simulink library "ctl_controller"  (R2016b)
settings: Solver=ode45  StartTime=0.0  StopTime=10.0  RelTol=1e-3  EnableMultiTasking=on
values from neighbouring files (symbols this model uses):
  ctl_ts = astrobee_fsw_step_size    [ctl_controller_init.m]
undefined symbols (not defined in the file or in its folder): astrobee_fsw_step_size, est_omega_B_ISS_B, est_V_B_ISS_ISS, tun_debug_ctl_use_truth
undefined symbols (not defined in the file): tun_truth_velocity_filt_cutoff_freq, tun_truth_velocity_filt_enable
libraries: math_utils x2, cex_control_executive_lib x1, clc_closed_loop_controller_lib x1, cmd_command_shaper_lib x1, simulink x1
settings Model: Creator=mjmcinty  LastModifiedBy=jfusco1
settings DataIOCC: LimitDataPoints=on  SaveFormat=Array
settings OptimizationCC: LifeSpan=inf
settings DebuggingCC: SolverPrmCheckMsg=warning  AllowSymbolicDim=off  SFUnexpectedBacktrackingDiag=warning  SFNoUnconditionalDefaultTransitionDiag=warning  SFExecutionAtInitializationDiag=none
settings HardwareCC: ProdBitPerPointer=32  ProdBitPerSizeT=32  ProdBitPerPtrDiffT=32  ProdLargestAtomicFloat=None  ProdIntDivRoundTo=Undefined  ProdEndianess=Unspecified  ProdWordSize=32  ProdHWDeviceType=32-bit Generic
settings ModelReferenceCC: PropagateSignalLabelsOutOfModel=off
settings GRTTargetCC: TargetLangStandard=C89/C90 (ANSI)  GeneratePreprocessorConditionals=Disable all
settings ConfigComp: CovMetricSettings=dw  CovHtmlReporting=on  CovSaveCumulativeToWorkspaceVar=on  CovSaveSingleToWorkspaceVar=on  CovExternalEMLEnable=off  CovSFcnEnable=off

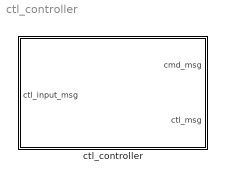
== system ctl_controller ==
  ctl_controller : Subsystem  TreatAsAtomicUnit=on  SystemSampleTime=ctl_ts

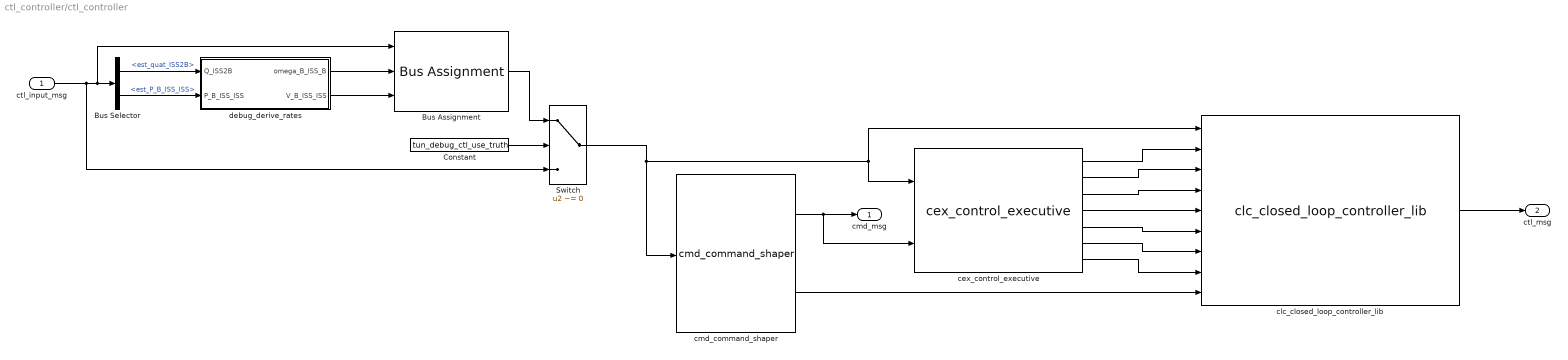
== system ctl_controller/ctl_controller ==
  ctl_input_msg : Inport  OutDataTypeStr=Bus: ctl_input_msg
  Bus Assignment : BusAssignment  AssignedSignals=est_omega_B_ISS_B,est_V_B_ISS_ISS
  Bus Selector : BusSelector  OutputSignals=est_quat_ISS2B,est_P_B_ISS_ISS
  Constant : Constant  Value=tun_debug_ctl_use_truth
  Switch : Switch  Criteria=u2 ~= 0
  cex_control_executive : cex_control_executive_lib/cex_control_executive
  clc_closed_loop_controller_lib : clc_closed_loop_controller_lib/clc_closed_loop_controller_lib
  cmd_command_shaper : cmd_command_shaper_lib/cmd_command_shaper
  debug_derive_rates : Subsystem
  cmd_msg : Outport
  ctl_msg : Outport  Port=2
  wires:
  ctl_input_msg/1 -> Switch/3, Bus Assignment/1, Bus Selector/1
  Bus Assignment/1 -> Switch/1
  Constant/1 -> Switch/2
  clc_closed_loop_controller_lib/1 -> ctl_msg/1
  cex_control_executive/5 -> clc_closed_loop_controller_lib/6
  cex_control_executive/4 -> clc_closed_loop_controller_lib/5
  cex_control_executive/3 -> clc_closed_loop_controller_lib/4
  cex_control_executive/2 -> clc_closed_loop_controller_lib/3
  cex_control_executive/1 -> clc_closed_loop_controller_lib/2
  cmd_command_shaper/1 -> cmd_msg/1, cex_control_executive/2
  Switch/1 -> cmd_command_shaper/1, cex_control_executive/1, clc_closed_loop_controller_lib/1
  cex_control_executive/6 -> clc_closed_loop_controller_lib/7
  cmd_command_shaper/2 -> clc_closed_loop_controller_lib/9
  cex_control_executive/7 -> clc_closed_loop_controller_lib/8
  Bus Selector/1 -> debug_derive_rates/1(Q_ISS2B)  "<est_quat_ISS2B>"
  Bus Selector/2 -> debug_derive_rates/2(P_B_ISS_ISS)  "<est_P_B_ISS_ISS>"
  debug_derive_rates/1(omega_B_ISS_B) -> Bus Assignment/2
  debug_derive_rates/2(V_B_ISS_ISS) -> Bus Assignment/3

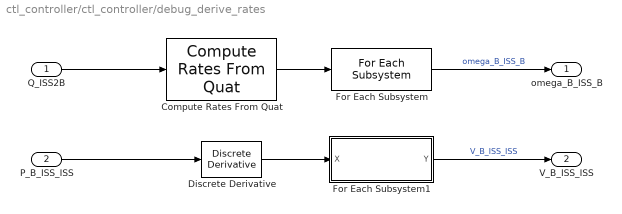
== system ctl_controller/ctl_controller/debug_derive_rates ==
  Q_ISS2B : Inport
  P_B_ISS_ISS : Inport  Port=2
  Compute Rates From Quat : math_utils/Compute Rates From Quat  SystemSampleTime=-1
  Discrete Derivative : simulink/Discrete/Discrete Derivative  gainval=1.0  ICPrevScaledInput=0.0  OutMin=[]  OutMax=[]  OutDataType=fixdt(1, 16)  OutScaling=2^-10  DoSatur=off
  For Each Subsystem : math_utils/For Each Subsystem  T=astrobee_fsw_step_size  omega=tun_truth_q_omega_filt_cutoff_freq  filt_enable=tun_truth_q_omega_filt_enable
  For Each Subsystem1 : Subsystem  TreatAsAtomicUnit=on  mask{T=astrobee_fsw_step_size, omega=tun_truth_velocity_filt_cutoff_freq, filt_enable=tun_truth_velocity_filt_enable}
      mask prompts: T "Sample Time:"; omega "Cutoff Freq (rad/sec):"; filt_enable "Enable Filter:"
      mask DialogControl DescTextVar Prompt: First Order Low Pass Discrete Time Filter
      mask Display: disp('1st Order Low-Pass');
  omega_B_ISS_B : Outport
  V_B_ISS_ISS : Outport  Port=2
  wires:
  P_B_ISS_ISS/1 -> Discrete Derivative/1
  Q_ISS2B/1 -> Compute Rates From Quat/1
  For Each Subsystem/1 -> omega_B_ISS_B/1  "omega_B_ISS_B"
  For Each Subsystem1/1(Y) -> V_B_ISS_ISS/1  "V_B_ISS_ISS"
  Compute Rates From Quat/1 -> For Each Subsystem/1
  Discrete Derivative/1 -> For Each Subsystem1/1(X)

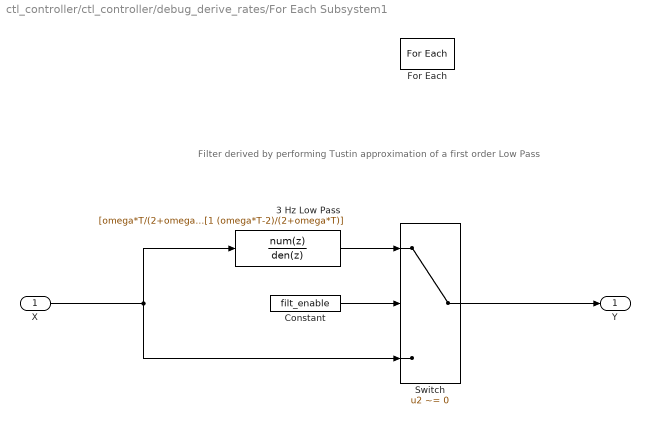
== system ctl_controller/ctl_controller/debug_derive_rates/For Each Subsystem1 ==
  note: Filter derived by performing Tustin approximation of a first order Low Pass
  X : Inport  Partition=on  PartitionDimension=1  PartitionWidth=1
  3 Hz Low Pass : DiscreteTransferFcn  Numerator=[omega*T/(2+omega*T) omega*T/(2+omega*T)]  Denominator=[1 (omega*T-2)/(2+omega*T)]  SampleTime=T
  Constant : Constant  Value=filt_enable
  For Each : ForEach  DisableCoverage=on  IndexMode=One-based
  Switch : Switch  Criteria=u2 ~= 0
  Y : Outport  ConcatenationDimension=1
  wires:
  Switch/1 -> Y/1
  X/1 -> 3 Hz Low Pass/1, Switch/3
  3 Hz Low Pass/1 -> Switch/1
  Constant/1 -> Switch/2
